simulink model "LKAS_AutoSave_20220223_1234"  (R2018b)
settings: Solver=FixedStepDiscrete  StartTime=0.0  StopTime=10.0  FixedStep=0.01  RelTol=1e-3
InitFcn:
  | tmpVer = ver('MATLAB');
  | tmpVer = str2num(tmpVer.Version);
  | % -------------------------------------------------------------------
  | %  MATLAB file generated by Simulink.saveVars on 21-Nov-2019 10:06:14
  | %  MATLAB version: 7.13.0.564 (R2011b)
  | % -------------------------------------------------------------------
  | 
  | 
  | SInt16 = Simulink.AliasType;
  | SInt16.Description = 'Num';
  | if (tmpVer > 7.11)
  | 	SInt16.DataScope = 'Auto';
  | end
  | SInt16.HeaderFile = 'Rte_Type.h';
  | SInt16.BaseType = 'int16';
  | 
  | SInt32 = Simulink.AliasType;
  | SInt32.Description = 'Num';
  | if (tmpVer > 7.11)
  | 	SInt32.DataScope = 'Auto';
  | end
  | SInt32.HeaderFile = 'Rte_Type.h';
  | SInt32.BaseType = 'int32';
  | 
  | SInt8 = Simulink.AliasType;
  | SInt8.Description = 'Num';
  | if (tmpVer > 7.11)
  | 	SInt8.DataScope = 'Auto';
  | end
  | SInt8.HeaderFile = 'Rte_Type.h';
  | SInt8.BaseType = 'int8';
  | 
  | T_A_m2_1024_1_u32 = Simulink.NumericType;
  | T_A_m2_1024_1_u32.Description = 'm2 (square meters  (m2))';
  | if (tmpVer > 7.11)
  | 	T_A_m2_1024_1_u32.DataScope = 'Auto';
  | end
  | T_A_m2_1024_1_u32.HeaderFile = 'Rte_Type.h';
  | T_A_m2_1024_1_u32.DataTypeMode = 'Fixed-point: slope and bias scaling';
  | T_A_m2_1024_1_u32.SignednessBool = false;
  | T_A_m2_1024_1_u32.WordLength = 32;
  | T_A_m2_1024_1_u32.FixedExponent = -10;
  | T_A_m2_1024_1_u32.SlopeAdjustmentFactor = 1;
  | T_A_m2_1024_1_u32.Bias = 0;
  | T_A_m2_1024_1_u32.DataTypeOverride = 'Inherit';
  | T_A_m2_1024_1_u32.IsAlias = true;
  | 
  | T_A_m2_65536_1_u16 = Simulink.NumericType;
  | T_A_m2_65536_1_u16.Description = 'm2 (square meters  (m2))';
  | if (tmpVer > 7.11)
  | 	T_A_m2_65536_1_u16.DataScope = 'Auto';
  | end
  | T_A_m2_65536_1_u16.HeaderFile = 'Rte_Type.h';
  | T_A_m2_65536_1_u16.DataTypeMode = 'Fixed-point: slope and bias scaling';
  | T_A_m2_65536_1_u16.SignednessBool = false;
  | T_A_m2_65536_1_u16.WordLength = 16;
  | T_A_m2_65536_1_u16.FixedExponent = -16;
  | T_A_m2_65536_1_u16.SlopeAdjustmentFactor = 1;
  | T_A_m2_65536_1_u16.Bias = 0;
  | T_A_m2_65536_1_u16.DataTypeOverride = 'Inherit';
  | ... (+4647 lines)
StopFcn:
  | clear  T_A_m2_1024_1_u32 T_A_m2_65536_1_u16 T_A_m2_Float32 T_A_mm2_10_1_u16 T_A_mm2_4_1_s16 T_A_mm2_Float32 T_Cnt_Num_10_1_u32 T_Cnt_Num_1_1_s16 T_Cnt_Num_1_1_s32 T_Cnt_Num_1_1_s8 T_Cnt_Num_1_1_u16 T_Cnt_Num_1_1_u32 T_Cnt_Num_1_1_u8 T_E_J_1_1_s32 T_E_J_Float32 T_E_kJ_128_1_s32 T_E_kJ_Float32 T_E_kwh_10_1_u16 T_E_kwh_Float32 T_Epl_kwhpkm_100_1_u16 T_Epl_kwhpkm_Float32 T_F_N_1_1_s16 T_F_N_Float32 T_I_A_1000_1_u16 T_I_A_1048576_1_s32 T_I_A_2048_1_s16 T_I_A_32_1_s16 T_I_A_Float32 T_I_mA_1_1_s16 T_I_mA_32768_128_s16 T_I_mA_Float32 T_J_kgpm2_128_1_u16 T_J_kgpm2_Float32 T_K_NA_1000_1_s16 T_K_NA_100_1_s16 T_K_NA_100_1_u16 T_K_NA_1024_1_s16 T_K_NA_1024_1_u16 T_K_NA_128_1_s16 T_K_NA_128_1_u16 T_K_NA_128_1_u8 T_K_NA_16777216_1_u32 T_K_NA_16_1_s16 T_K_NA_16_1_u16 T_K_NA_16_1_u8 T_K_NA_1_16_u16 T_K_NA_1_1_s16 T_K_NA_1_1_u16 T_K_NA_1_1_u8 T_K_NA_32768_1_s16 T_K_NA_32768_1_u16 T_K_NA_32_1_s8 T_K_NA_4096_1_u16 T_K_NA_4194304_1_s32 T_K_NA_4194304_1_u16 T_K_NA_65536_1_s32 T_K_NA_65536_1_u16 T_K_NA_8192_1_s16 T_K_NA_8_1_s16 T_K_NA_Float32 T_M_Nm_16_1_s16 T_M_Nm_1_1_s16 T_M_Nm_32768_1_s16 T_M_Nm_32_1_s16 T_M_Nm_4_1_s16 T_M_Nm_512_1_s16 T_M_Nm_Float32 T_P_W_1_4_s16 T_P_W_1_8_s16 T_P_W_Float32 T_P_kW_128_1_s16 T_P_kW_1_8_s16 T_P_kW_8_1_s32 T_P_kW_Float32 T_Pct_pct_1024_1_s32 T_Pct_pct_1024_1_u32 T_Pct_pct_10_1_s16 T_Pct_pct_10_1_u32 T_Pct_pct_128_100_s8 T_Pct_pct_1_1_s16 T_Pct_pct_1_4_u8 T_Pct_pct_255_100_u16 T_Pct_pct_255_100_u8 T_Pct_pct_256_1_s16 T_Pct_pct_256_1_u16 T_Pct_pct_65535_100_u16 T_Pct_pct_Float32 T_R_ohm_1024_1_s16 T_R_ohm_32_1_s16 T_R_ohm_Float32 T_TK_K_16_1_s16 T_TK_K_Float32 T_T_degC_10_400_1_u16 T_T_degC_16_1_s16 T_T_degC_1_40_1_u8 T_T_degC_2_80_1_u8 T_T_degC_Float32 T_U_V_1000_1_u16 T_U_V_10_1_u8 T_U_V_200_1_u8 T_U_V_32_1_s16 T_U_V_4096_1_s16 T_U_V_512_1_s16 T_U_V_65535_8_u16 T_U_V_8192_1_u16 T_U_V_Float32 T_U_mV_1_1_s16 T_U_mV_256_20_u16 T_U_mV_Float32 T_V_l_256_1_s16 T_V_l_4096_1_s16 T_V_l_64_1_s16 T_V_l_65535_100_u16 T_V_l_Float32 T_V_ml_128_1_s16 T_V_ml_1_1_s16 T_V_ml_32768_1_s16 T_V_ml_Float32 T_V_ul_32_1_u16 T_V_ul_Float32 T_Vpl_clpkm_512_1_u16 T_Vpl_clpkm_Float32 T_a_kphps_16_1_s16 T_a_kphps_Float32 T_a_mps2_128_1_s16 T_a_mps2_Float32 T_c_MJpkg_256_1_s16 T_c_MJpkg_Float32 T_c_kJpgpK_1024_1_s16 T_c_kJpgpK_Float32 T_c_kJpkgpK_128_1_u16 T_c_kJpkgpK_Float32 T_chrg_Ah_1_1_s16 T_chrg_Ah_1_1_u16 T_chrg_Ah_1_1_u8 T_chrg_Ah_256_1_u16 T_chrg_Ah_4194304_1_s32 T_chrg_Ah_512_1_u16 T_chrg_Ah_8_1_u16 T_chrg_Ah_Float32 T_cmp_NA_100_1_s16 T_cmp_NA_128_1_s16 T_cmp_NA_16_1_s16 T_cmp_NA_32768_1_u16 T_cmp_NA_Float32 T_d2n_rpmps2_4_1_s16 T_d2n_rpmps2_Float32 T_dPct_pctps_16_1_s16 T_dPct_pctps_256_1_s16 T_dPct_pctps_Float32 T_dT_degCps_128_1_s16 T_dT_degCps_Float32 T_dV_lph_1_1_s16 T_dV_lph_Float32 T_dV_lpm_128_1_s16 T_dV_lpm_32_1_s16 T_dV_lpm_Float32 T_dV_lps_1024_1_u16 T_dV_lps_4_1_u16 T_dV_lps_Float32 T_dV_mlps_1024_1_s16 T_dV_mlps_Float32 T_d_BitField16 T_dm_gps_128_1_s16 T_dm_gps_128_1_u16 T_dm_gps_256_1_u16 T_dm_gps_Float32 T_dm_mgps_1_1_s16 T_dm_mgps_Float32 T_dn_rpmps_1_1_s16 T_dn_rpmps_2_1_s16 T_dn_rpmps_Float32 T_dp_Paps_1_1_s16 T_dp_Paps_Float32 T_dp_kPaps_1_1_s16 T_dp_kPaps_8_1_s16 T_dp_kPaps_Float32 T_dphi_degps_128_1_s16 T_dphi_degps_8_1_s16 T_dphi_degps_Float32 T_dr_ps_256_1_s16 T_dr_ps_Float32 T_drho_mgplps_1_2_s16 T_drho_mgplps_Float32 T_e_NA_1_1_u8 T_f_Hz_1_1_u16 T_f_Hz_1_1_u32 T_f_Hz_64_1_u16 T_f_Hz_8_1_s16 T_f_Hz_Float32 T_g_BitField32 T_l_km_16_1_s16 T_l_km_1_1_u16 T_l_km_1_1_u32 T_l_km_Float32 T_l_m_1024_1_s16 T_l_m_16_1_s16 T_l_m_1_1_u32 T_l_m_Float32 T_l_mm_16_1_s16 T_l_mm_1_1_u16 T_l_mm_4096_1_s16 T_l_mm_4_1_u8 T_l_mm_64_1_s16 T_l_mm_Float32 T_m_g_1_1_s16 T_m_g_2048_1_s16 T_m_g_32_1_u16 T_m_g_Float32 T_m_kg_1024_1_s16 T_m_kg_1_1_s16 T_m_kg_1_1_u32 T_m_kg_Float32 T_m_mg_128_1_s16 T_m_mg_32_1_s16 T_m_mg_Float32 T_n_rpm_1_1_s16 T_n_rpm_1_25_u8 T_n_rpm_256_50_u16 T_n_rpm_2_25_u8 T_n_rpm_4_1_u16 T_n_rpm_Float32 T_p_MPa_64_1_s16 T_p_MPa_Float32 T_p_Pa_1_1_s16 T_p_Pa_Float32 T_p_kPa_1_10_u16 T_p_kPa_1_1_s16 T_p_kPa_1_1_u8 T_p_kPa_256_1_u16 T_p_kPa_32_1_u16 T_p_kPa_64_1_s16 T_p_kPa_Float32 T_phi_deg_100_1_s16 T_phi_deg_1024_1_s16 T_phi_deg_128_1_s16 T_phi_deg_1_1_u8 T_phi_deg_256_1_s16 T_phi_deg_2_1_s8 T_phi_deg_32_1_s16 T_phi_deg_512_6_s32 T_phi_deg_Float32 T_phi_rad_2048_1_s16 T_phi_rad_Float32 T_r_NA_1024_1_s16 T_r_NA_1024_1_u16 T_r_NA_16384_1_s16 T_r_NA_16_1_s16 T_r_NA_256_1_s8 T_r_NA_256_1_u16 T_r_NA_32768_1_u16 T_r_NA_32_1_u16 T_r_NA_4096_1_s16 T_r_NA_65535_2_u16 T_r_NA_8192_1_u16 T_r_NA_Float32 T_rho_gpl_8192_1_s16 T_rho_gpl_Float32 T_rho_kgpm3_16_1_s16 T_rho_kgpm3_Float32 T_rho_mgpl_1_1_s16 T_rho_mgpl_64_1_s16 T_rho_mgpl_Float32 T_t_hour_1_1_s16 T_t_hour_Float32 T_t_m_1_1_u16 T_t_m_Float32 T_t_ms_1_1_s16 T_t_ms_1_1_u16 T_t_ms_1_1_u32 T_t_ms_4096_1_s16 T_t_ms_64_1_s16 T_t_ms_Float32 T_t_s_1000_1_s16 T_t_s_100_1_s16 T_t_s_10_1_s16 T_t_s_10_1_u16 T_t_s_1_1_s16 T_t_s_1_1_u16 T_t_s_1_1_u32 T_t_s_Float32 T_t_us_10_1_u32 T_t_us_1_1_s16 T_t_us_1_1_u32 T_t_us_1_4_u16 T_t_us_Float32 T_v_kph_1_1_u8 T_v_kph_64_1_s16 T_v_kph_64_1_u16 T_v_kph_Float32 T_v_mps_256_1_s16 T_v_mps_Float32 T_w_radps_32_1_s16 T_w_radps_Float32 T_y_BitField8 T_y_BitFieldDiagProgress T_y_BitFieldDiagStatus T_y_NA_1_1_u8 SInt16 SInt32 SInt8 T_BOOLEAN UInt16 UInt32 UInt8 s16 s32 s8 u16 u32 u8
model workspace (MAT data in the model file):
  MCOS : class17 (value not decoded)
  MCOS : class17 (value not decoded)
  MCOS : class17 (value not decoded)
  MCOS : class17 (value not decoded)
  MCOS : class17 (value not decoded)
  MCOS : class17 (value not decoded)
  MCOS : class17 (value not decoded)
  MCOS : class17 (value not decoded)
  MCOS : class17 (value not decoded)
  MCOS : class17 (value not decoded)
  MCOS : class17 (value not decoded)
  MCOS : class17 (value not decoded)
  MCOS : class17 (value not decoded)
  MCOS : class17 (value not decoded)
  MCOS : class17 (value not decoded)
  MCOS : class17 (value not decoded)
  MCOS : class17 (value not decoded)
  MCOS : class17 (value not decoded)
  MCOS : class17 (value not decoded)
  MCOS : class17 (value not decoded)
  MCOS : class17 (value not decoded)
  MCOS : class17 (value not decoded)
  MCOS : class17 (value not decoded)
  MCOS : class17 (value not decoded)
  MCOS : class17 (value not decoded)
  MCOS : class17 (value not decoded)
  MCOS : class17 (value not decoded)
  MCOS : class17 (value not decoded)
  MCOS : class17 (value not decoded)
  MCOS : class17 (value not decoded)
  MCOS : class17 (value not decoded)
  MCOS : class17 (value not decoded)
  MCOS : class17 (value not decoded)
  MCOS : class17 (value not decoded)
  MCOS : class17 (value not decoded)
  MCOS : class17 (value not decoded)
  MCOS : class17 (value not decoded)
  MCOS : class17 (value not decoded)
  MCOS : class17 (value not decoded)
  MCOS : class17 (value not decoded)
  MCOS : class17 (value not decoded)
  MCOS : class17 (value not decoded)
  MCOS : class17 (value not decoded)
  MCOS : class17 (value not decoded)
  MCOS : class17 (value not decoded)
  MCOS : class17 (value not decoded)
  MCOS : class17 (value not decoded)
  MCOS : class17 (value not decoded)
  MCOS : class17 (value not decoded)
  MCOS : class17 (value not decoded)
  MCOS : class17 (value not decoded)
  MCOS : class17 (value not decoded)
  MCOS : class17 (value not decoded)
  MCOS : class17 (value not decoded)
  MCOS : class17 (value not decoded)
  MCOS : class17 (value not decoded)
  MCOS : class17 (value not decoded)
  MCOS : class17 (value not decoded)
  MCOS : class17 (value not decoded)
  MCOS : class17 (value not decoded)
  MCOS : class17 (value not decoded)
  MCOS : class17 (value not decoded)
  MCOS : class17 (value not decoded)
  MCOS : class17 (value not decoded)
  MCOS : class17 (value not decoded)
  MCOS : class17 (value not decoded)
  MCOS : class17 (value not decoded)
  MCOS : class17 (value not decoded)
  MCOS : class17 (value not decoded)
  MCOS : class17 (value not decoded)
  MCOS : class17 (value not decoded)
  MCOS : class17 (value not decoded)
  MCOS : class17 (value not decoded)
  MCOS : class17 (value not decoded)
  MCOS : class17 (value not decoded)
  MCOS : class17 (value not decoded)
  MCOS : class17 (value not decoded)
  MCOS : class17 (value not decoded)
  MCOS : class17 (value not decoded)
  MCOS : class17 (value not decoded)
  MCOS : class17 (value not decoded)
  MCOS : class17 (value not decoded)
  MCOS : class17 (value not decoded)
  MCOS : class17 (value not decoded)
  MCOS : class17 (value not decoded)
  MCOS : class17 (value not decoded)
  MCOS : class17 (value not decoded)
  MCOS : class17 (value not decoded)
  MCOS : class17 (value not decoded)
  MCOS : class17 (value not decoded)
  MCOS : class17 (value not decoded)
  MCOS : class17 (value not decoded)
  MCOS : class17 (value not decoded)
  MCOS : class17 (value not decoded)
  MCOS : class17 (value not decoded)
  MCOS : class17 (value not decoded)
  MCOS : class17 (value not decoded)
  MCOS : class17 (value not decoded)
  MCOS : class17 (value not decoded)
  MCOS : class17 (value not decoded)
  MCOS : class17 (value not decoded)
  MCOS : class17 (value not decoded)
undefined symbols (not defined in the file): LKA_CarWidth, LKA_SampleTime, LKA_StrRatio_C, LKA_Veh2CamL_C, LKA_Veh2CamW_C, LKA_WhlBaseL_C, LL_CompHdAg_C, LL_CompSWA_C, LL_CrvtPrvwT_C, LL_DesDvt_C, LL_DvtComp_C, LL_DvtPrvwT_C, LL_DvtSpdDet_vDvtSpdMin_C, LL_HandsOff_ExitTime, LL_HandsOff_TextTime, LL_HandsOff_WarnTime, LL_HdAgExT_C, LL_HdAgPrvwT_C, LL_LAccMax_C, LL_LAccRMax_C, LL_LDW_EarliestWarnLine_C, LL_LDW_LatestWarnLine_C, LL_LDWS_SUPPRESS_HEADING, LL_LFClb_TFC_FfCtlRatio_C, LL_LFClb_TFC_KdBalance_C, LL_LFClb_TFC_KdMaxSWA_C, LL_LFClb_TFC_KdV1_C, LL_LFClb_TFC_KdV2_C, LL_LFClb_TFC_KdVehSpdLwr_C, LL_LFClb_TFC_KdVehSpdUpr_C, LL_LFClb_TFC_Ki_C, LL_LFClb_TFC_KiMaxSWA_C, LL_LFClb_TFC_Kp_C, LL_LFClb_TFC_KpKlat_C, LL_LFClb_TFC_KpV1_C, LL_LFClb_TFC_KpV2_C, LL_LFClb_TFC_KpVehSpdLwr_C, LL_LFClb_TFC_KpVehSpdUpr_C, LL_LFClb_TFC_PrvwT_C, LL_LKA_EarliestWarnLine_C, LL_LKA_LatestWarnLine_C, LL_LKAExPrcs_ExitC0Dvt, LL_LKAExPrcs_ExitC0Swt, LL_LKAExPrcs_tiExitTime1, LL_LKAExPrcs_tiExitTime2, LL_LKAExPrcs_tiExitTime3, LL_LKAS_OUT_OF_CONTROL_LAT_VEL, LL_LKAS_OUT_OF_CONTROL_TTLC, LL_LKASWASyn_M0, LL_LKASWASyn_M1, LL_LKASWASyn_M2, LL_LKASWASyn_M3K, LL_LKASWASyn_SWAaddMax, LL_LKASWASyn_T2, LL_LKASWASyn_tiTrqSwaRtTime, LL_LKASWASyn_tiTrqSwaTime, LL_LKASWASyn_TrqMax, LL_LKASWASyn_TrqSwaAddSwt, LL_LKASWASyn_TrqSwaRateDiff, LL_LSpdCompT_C ... (+43)
libraries: simulink x138, canmsglib x8, dspstat3 x3, simulink_extras x1
(part 10 of 20)

== system LKAS_AutoSave_20220223_1234/LKAS/LL/LLOn/LKA/Lane Following (LF)/Preview Information Calculation (PIC) ==
  PIC_bsLKAInPInfo : Inport
  Bus Creator : BusCreator  Inputs=6
  Bus Selector1 : BusSelector  OutputSignals=bsPrDvtInfo.lPrvwDvtMean,bsPrHdAgInfo.phiPrvwHdAgMean,bsPrCrvtInfo.crPrvwCrvtMean,LaneWidth,bsPrHdAgInfo.PrvwZMean,bsPrCrvtInfo.crPrvwCrvtMean
  PIC_bsPrvwInfo : Outport
  wires:
  Bus Selector1/4 -> Bus Creator/4  "<LaneWidth>"
  Bus Creator/1 -> PIC_bsPrvwInfo/1
  PIC_bsLKAInPInfo/1 -> Bus Selector1/1
  Bus Selector1/3 -> Bus Creator/3  "<crPrvwCrvtMean>"
  Bus Selector1/2 -> Bus Creator/2  "<phiPrvwHdAgMean>"
  Bus Selector1/1 -> Bus Creator/1  "<lPrvwDvtMean>"
  Bus Selector1/5 -> Bus Creator/5  "<PrvwZMean>"
  Bus Selector1/6 -> Bus Creator/6  "<crPrvwCrvtMean>"

== system LKAS_AutoSave_20220223_1234/LKAS/LL/LLOn/LKA/Lane Following (LF)/Trajectory Following Control (TFC) ==
  TFC_bsPrvwInfo : Inport
  TFC_bsInInfoSyn : Inport  Port=2
  TFC_bsTFCClb : Inport  Port=3
  Bus Selector1 : BusSelector  OutputSignals=bsLKAClb.LL_TFCClb.LL_LFClb_TFC_PrvwT_C,bsLKAClb.LL_TFCClb.LL_LFClb_TFC_KpKlat_C,bsLKAClb.LL_TFCClb.LL_LFClb_TFC_KpVehSpdLwr_C,bsLKAClb.LL_TFCClb.LL_LFClb_TFC_KpVehSpdUpr_C,bsLKAClb.LL_TFCClb.LL_LFClb_TFC_KpV1_C,bsLKAClb.LL_TFCClb.LL_LFClb_TFC_KpV2_C,bsLKAClb.LL_TFCClb.LL_LFClb_TFC_Kp_C,bsLKAClb.LL_TFCClb.LL_LFClb_TFC_KiMaxSWA_C,bsLKAClb.LL_TFCClb.LL_LFClb_TFC_Ki_C,bsLKAClb.LL_TFCClb.LL_LFClb_TFC_KdMaxSWA_C,bsLKAClb.LL_TFCClb.LL_LFClb_TFC_KdBalance_C,bsLKAClb.LL_TFCClb.LL_LFClb_TFC_KdVehSpdLwr_C,bsLKAClb.LL_TFCClb.LL_LFClb_TFC_KdVehSpdUpr_C,bsLKAClb.LL_TFCClb.LL_LFClb_TFC_KdV1_C,bsLKAClb.LL_TFCClb.LL_LFClb_TFC_KdV2_C,bsConstantClb.LKA_CarWidth,bsLKAClb.LL_TFCClb.LL_LFClb_TFC_FfCtlRatio_C,bsConstantClb.LKA_WhlBaseL_C,bsConstantClb.LKA_StrRatio_C
  Bus Selector2 : BusSelector  OutputSignals=lPrvwDvtMean (signal 1),phiPrvwHdAgMean (signal 2),crPrvwCrvtMean (signal 3),LaneWidth (signal 4),PrvwZMean (signal 5),crPrvwCrvtMean (signal 6)
  Bus Selector3 : BusSelector  OutputSignals=bsLaneInfo.bsL0Info,bsLaneInfo.bsR0Info,bsVehMovInfo.ESC_VehSpd
  Feedback Control (FbCtl) : Subsystem
  Feedforward Control (FfCtl) : Subsystem
  TFC_phiFfSWACmd : Outport
  TFC_phiPropSWACmd : Outport  Port=2
  TFC_phiIntegSWACmd : Outport  Port=3
  TFC_phiDiffSWACmd : Outport  Port=4
  wires:
  Bus Selector1/16 -> Feedback Control (FbCtl)/25(FbCtl_CarWidth)  "<LKA_CarWidth>"
  Bus Selector2/4 -> Feedback Control (FbCtl)/7(FbCtl_LaneWidth)  "<LaneWidth (signal 4)>"
  Bus Selector1/15 -> Feedback Control (FbCtl)/24(FbCtl_KdV2_C)  "<LL_LFClb_TFC_KdV2_C>"
  Bus Selector1/14 -> Feedback Control (FbCtl)/23(FbCtl_KdV1_C)  "<LL_LFClb_TFC_KdV1_C>"
  Bus Selector1/13 -> Feedback Control (FbCtl)/22(FbCtl_KdVehSpdUpr_C)  "<LL_LFClb_TFC_KdVehSpdUpr_C>"
  Bus Selector1/12 -> Feedback Control (FbCtl)/21(FbCtl_KdVehSpdLwr_C)  "<LL_LFClb_TFC_KdVehSpdLwr_C>"
  Bus Selector1/7 -> Feedback Control (FbCtl)/16(FbCtl_Kp_C)  "<LL_LFClb_TFC_Kp_C>"
  Feedback Control (FbCtl)/3(FbCtl_phiFbDiffCtlSWA) -> TFC_phiDiffSWACmd/1
  Bus Selector3/2 -> Feedback Control (FbCtl)/2(FbCtl_bsR0Info)  "<bsR0Info>"
  Bus Selector3/1 -> Feedback Control (FbCtl)/1(FbCtl_bsL0Info)  "<bsL0Info>"
  TFC_bsInInfoSyn/1 -> Bus Selector3/1
  Bus Selector2/3 -> Feedforward Control (FfCtl)/3(FfCtl_crPrvwCrvt), Feedback Control (FbCtl)/6(FbCtl_PrvwCrvt)  "<crPrvwCrvtMean (signal 3)>"
  Feedforward Control (FfCtl)/1(FfCtl_phiFfSWA) -> TFC_phiFfSWACmd/1  "phiFfSWA"
  Feedback Control (FbCtl)/1(FbCtl_phiFbPropCtlSWA) -> TFC_phiPropSWACmd/1
  TFC_bsPrvwInfo/1 -> Bus Selector2/1  "bsPrvwInfo"
  Bus Selector2/1 -> Feedback Control (FbCtl)/4(FbCtl_PrvwDvt)  "<lPrvwDvtMean (signal 1)>"
  TFC_bsTFCClb/1 -> Bus Selector1/1
  Bus Selector1/1 -> Feedback Control (FbCtl)/10(FbCtl_PrvwT_C)  "<LL_LFClb_TFC_PrvwT_C>"
  Bus Selector1/2 -> Feedback Control (FbCtl)/11(FbCtl_KpKlat_C)  "<LL_LFClb_TFC_KpKlat_C>"
  Bus Selector3/3 -> Feedforward Control (FfCtl)/2(FfCtl_vVehSpd), Feedback Control (FbCtl)/3(FbCtl_VehSpd)  "<ESC_VehSpd>"
  Bus Selector1/3 -> Feedback Control (FbCtl)/12(FbCtl_KpVehSpdLwr_C)  "<LL_LFClb_TFC_KpVehSpdLwr_C>"
  Bus Selector1/4 -> Feedback Control (FbCtl)/13(FbCtl_KpVehSpdUpr_C)  "<LL_LFClb_TFC_KpVehSpdUpr_C>"
  Bus Selector1/5 -> Feedback Control (FbCtl)/14(FbCtl_KpV1_C1)  "<LL_LFClb_TFC_KpV1_C>"
  Bus Selector1/6 -> Feedback Control (FbCtl)/15(FbCtl_KpV2_C1)  "<LL_LFClb_TFC_KpV2_C>"
  Bus Selector1/17 -> Feedforward Control (FfCtl)/1(FfCtl_FfCtlRatio_C)  "<LL_LFClb_TFC_FfCtlRatio_C>"
  Bus Selector1/8 -> Feedback Control (FbCtl)/17(FbCtl_KiMaxSWA_C)  "<LL_LFClb_TFC_KiMaxSWA_C>"
  Bus Selector1/9 -> Feedback Control (FbCtl)/18(FbCtl_Ki_C)  "<LL_LFClb_TFC_Ki_C>"
  Feedback Control (FbCtl)/2(FbCtl_phiFbIntegCtlSWA) -> TFC_phiIntegSWACmd/1
  Bus Selector1/10 -> Feedback Control (FbCtl)/19(FbCtl_KdMaxSWA)  "<LL_LFClb_TFC_KdMaxSWA_C>"
  Bus Selector1/11 -> Feedback Control (FbCtl)/20(FbCtl_KdBalance)  "<LL_LFClb_TFC_KdBalance_C>"
  Bus Selector1/18 -> Feedforward Control (FfCtl)/4(FfCtl_lWhlBase_SY)  "<LKA_WhlBaseL_C>"
  Bus Selector1/19 -> Feedforward Control (FfCtl)/5(FfCtl_rTraRatio_C)  "<LKA_StrRatio_C>"
  Bus Selector2/2 -> Feedback Control (FbCtl)/5(FbCtl_PrvwHdAg)  "<phiPrvwHdAgMean (signal 2)>"
  Bus Selector2/5 -> Feedback Control (FbCtl)/8(PrvwZMean)  "<PrvwZMean (signal 5)>"
  Bus Selector2/6 -> Feedback Control (FbCtl)/9(PrvwCrvtMean)  "<crPrvwCrvtMean (signal 6)>"

== system LKAS_AutoSave_20220223_1234/LKAS/LL/LLOn/LKA/Plan To LaneFollowing (PTLF)/InsideJudge ==
  Flg : Inport
  Crvt : Inport  Port=2
  Compare To Constant : simulink/Logic and Bit Operations/Compare To Constant  relop===  const=1  OutDataTypeStr=boolean
  Compare To Constant1 : simulink/Logic and Bit Operations/Compare To Constant  relop===  const=2  OutDataTypeStr=boolean
  Constant : Constant  Value=0.001  OutDataTypeStr=single
  Constant3 : Constant  Value=-0.001  OutDataTypeStr=single
  Logical Operator : Logic  AllPortsSameDT=off  OutDataTypeStr=boolean
  Logical Operator1 : Logic  AllPortsSameDT=off  OutDataTypeStr=boolean
  Logical Operator2 : Logic  Operator=OR  AllPortsSameDT=off  OutDataTypeStr=boolean
  Relational Operator : RelationalOperator  OutDataTypeStr=boolean  RndMeth=Simplest
  Relational Operator1 : RelationalOperator  Operator=<=  OutDataTypeStr=boolean  RndMeth=Simplest
  Out1 : Outport
  wires:
  Compare To Constant/1 -> Logical Operator1/1  "LeftActive"
  Logical Operator1/1 -> Logical Operator2/1
  Logical Operator/1 -> Logical Operator2/2
  Flg/1 -> Compare To Constant1/1, Compare To Constant/1
  Relational Operator/1 -> Logical Operator/2  "RightCrvt"
  Compare To Constant1/1 -> Logical Operator/1  "RightActive"
  Constant/1 -> Relational Operator/2
  Relational Operator1/1 -> Logical Operator1/2  "LeftCrvt"
  Constant3/1 -> Relational Operator1/2
  Logical Operator2/1 -> Out1/1
  Crvt/1 -> Relational Operator1/1, Relational Operator/1

== system LKAS_AutoSave_20220223_1234/LKAS/LL/LLOn/LKA/Plan To LaneFollowing (PTLF)/InsideJudge1 ==
  Flg : Inport
  HdAgLft : Inport  Port=2
  HdAgRgt : Inport  Port=3
  T1 : Inport  Port=4
  Plan : Inport  Port=5
  Time : Inport  Port=6
  If : If  IfExpression=u1 == 1  ElseIfExpressions=u1 == 2
  If Action Subsystem : Subsystem  TreatAsAtomicUnit=on
  If Action Subsystem1 : Subsystem  TreatAsAtomicUnit=on
  If Action Subsystem2 : Subsystem  TreatAsAtomicUnit=on
  Merge : Merge  Inputs=3  InitialOutput=1
  Merge1 : Merge  Inputs=3  InitialOutput=0
  T1_1 : Outport
  Plan_1 : Outport  Port=2
  wires:
  Flg/1 -> If/1
  If/1 -> If Action Subsystem/Action
  If/2 -> If Action Subsystem1/Action
  If/3 -> If Action Subsystem2/Action
  HdAgLft/1 -> If Action Subsystem/3(HdAgLft)
  If Action Subsystem/1(T1_1) -> Merge/1
  If Action Subsystem1/1(T1_1) -> Merge/2
  If Action Subsystem2/1(T1_1) -> Merge/3
  If Action Subsystem/2(Plan_1) -> Merge1/1
  If Action Subsystem1/2(Plan_1) -> Merge1/2
  If Action Subsystem2/2(Plan_1) -> Merge1/3
  T1/1 -> If Action Subsystem/1(T1), If Action Subsystem1/1(T1), If Action Subsystem2/1(T1)
  Plan/1 -> If Action Subsystem/2(Plan), If Action Subsystem1/2(Plan), If Action Subsystem2/2(Plan)
  HdAgRgt/1 -> If Action Subsystem1/3(HdAgRgt)
  Merge/1 -> T1_1/1
  Merge1/1 -> Plan_1/1
  Time/1 -> If Action Subsystem1/4(Time), If Action Subsystem/4(Time)

== system LKAS_AutoSave_20220223_1234/LKAS/LL/LLOn/LKA/Plan To LaneFollowing (PTLF)/LowPass ==
  T : Inport
  u : Inport  Port=2
  dT : Inport  Port=3
  Add : Sum  Inputs=+-
  Add1 : Sum
  Add2 : Sum  OutDataTypeStr=single
  Divide : Product  Inputs=*/
  Divide1 : Product  Inputs=**
  Memory3 : Memory  InheritSampleTime=on
  SWACmdSyn_tiSmplT_C4 : Constant  OutDataTypeStr=single
  Saturation : Saturate  UpperLimit=50  LowerLimit=0
      settings: AttributesFormatString="Min = %<LowerLimit>  Max = %<UpperLimit>"
  Switch : Switch  Criteria=u2 > Threshold  Threshold=30
  Unit Delay : UnitDelay  SampleTime=-1
  y : Outport
  wires:
  Switch/1 -> Unit Delay/1, y/1
  Memory3/1 -> Add2/2
  Saturation/1 -> Memory3/1, Switch/2
  Add2/1 -> Saturation/1
  SWACmdSyn_tiSmplT_C4/1 -> Add2/1
  Add1/1 -> Switch/1
  Unit Delay/1 -> Add1/2, Add/2
  Divide1/1 -> Add1/1
  Add/1 -> Divide1/2
  Divide/1 -> Divide1/1
  u/1 -> Add/1, Switch/3
  dT/1 -> Divide/1
  T/1 -> Divide/2

== system LKAS_AutoSave_20220223_1234/LKAS/LL/LLOn/LKA/Plan To LaneFollowing (PTLF)/TickTime (TTime) ==
  Add2 : Sum  OutDataTypeStr=single
  Memory3 : Memory  InheritSampleTime=on
  Saturation : Saturate  UpperLimit=50  LowerLimit=0
      settings: AttributesFormatString="Min = %<LowerLimit>  Max = %<UpperLimit>"
  Out1 : Outport
  wires:
  Add2/1 -> Saturation/1
  Memory3/1 -> Add2/2
  Saturation/1 -> Out1/1, Memory3/1
  [LKA_SampleTime] -> Add2/1

== system LKAS_AutoSave_20220223_1234/LKAS/LL/LLOn/LKA/Plan To LaneFollowing (PTLF)/TimeGain ==
  Time : Inport
  T1 : Inport  Port=2
  TFC : Inport  Port=3
  Add1 : Sum
  Add2 : Sum  Inputs=+-
  Add3 : Sum  Inputs=-+
  Constant1 : Constant  Value=0  OutDataTypeStr=single
  Constant4 : Constant  OutDataTypeStr=single
  Divide : Product  Inputs=*/
  Divide8 : Product  Inputs=**
  Saturation4 : Saturate  UpperLimit=1  LowerLimit=0
      settings: AttributesFormatString="Min = %<LowerLimit>  Max = %<UpperLimit>"
  Out1 : Outport
  wires:
  Saturation4/1 -> Divide8/2
  Constant1/1 -> Add1/1, Add3/1
  Divide8/1 -> Add1/2
  Add1/1 -> Out1/1
  TFC/1 -> Divide/2
  T1/1 -> Add2/2
  Time/1 -> Add2/1
  Divide/1 -> Saturation4/1
  Add2/1 -> Divide/1
  Constant4/1 -> Add3/2
  Add3/1 -> Divide8/1

== system LKAS_AutoSave_20220223_1234/LKAS/LL/LLOn/LKA Input Processing (LKAInP)/Deviation Calculation (Dvt)/Left Front Conner Deviation Calculation (LFCDvtCalc) ==
  LFCDvtCalc_bsHdAgInfo : Inport
  LFCDvtCalc_lDvt : Inport  Port=2
  LFCDvtCalc_bsLLClb : Inport  Port=3
  Add1 : Sum  OutDataTypeStr=single
  Add5 : Sum  OutDataTypeStr=single
  Bus Selector : BusSelector  OutputSignals=bsConstantClb.LKA_Veh2CamW_C,bsConstantClb.LKA_Veh2CamL_C
  Cos2 : Trigonometry  Operator=cos
  Divide : Product  Inputs=**
  Divide1 : Product  Inputs=**
  Gain1 : Gain  Gain=-1  OutDataTypeStr=single
  Sin : Trigonometry
  DvtCalc_lLftDvt : Outport
  wires:
  LFCDvtCalc_lDvt/1 -> Add1/1
  Bus Selector/1 -> Add1/2  "<LKA_Veh2CamW_C>"
  LFCDvtCalc_bsLLClb/1 -> Bus Selector/1
  Bus Selector/2 -> Divide1/1  "<LKA_Veh2CamL_C>"
  LFCDvtCalc_bsHdAgInfo/1 -> Cos2/1, Sin/1
  Gain1/1 -> DvtCalc_lLftDvt/1
  Cos2/1 -> Divide/2
  Sin/1 -> Divide1/2
  Divide/1 -> Add5/1
  Divide1/1 -> Add5/2
  Add1/1 -> Divide/1
  Add5/1 -> Gain1/1

== system LKAS_AutoSave_20220223_1234/LKAS/LL/LLOn/LKA Input Processing (LKAInP)/Deviation Calculation (Dvt)/Right Front Conner Deviation Calculation (RFCDvtCalc) ==
  RFCDvtCalc_lDvt : Inport
  RFCDvtCalc_bsHdAgInfo : Inport  Port=2
  RFCDvtCalc_bsLLClb : Inport  Port=3
  Add1 : Sum  Inputs=+-  OutDataTypeStr=single
  Add5 : Sum  OutDataTypeStr=single
  Bus Selector1 : BusSelector  OutputSignals=bsConstantClb.LKA_Veh2CamW_C,bsConstantClb.LKA_Veh2CamL_C
  Cos2 : Trigonometry  Operator=cos
  Divide : Product  Inputs=**
  Divide1 : Product  Inputs=**
  Sin : Trigonometry
  DvtCalc_lRgtDvt : Outport
  wires:
  RFCDvtCalc_lDvt/1 -> Add1/1
  Bus Selector1/1 -> Add1/2  "<LKA_Veh2CamW_C>"
  Bus Selector1/2 -> Divide1/1  "<LKA_Veh2CamL_C>"
  Add5/1 -> DvtCalc_lRgtDvt/1
  Sin/1 -> Divide1/2
  Divide1/1 -> Add5/2
  RFCDvtCalc_bsHdAgInfo/1 -> Cos2/1, Sin/1
  Cos2/1 -> Divide/2
  Add1/1 -> Divide/1
  Divide/1 -> Add5/1
  RFCDvtCalc_bsLLClb/1 -> Bus Selector1/1

== system LKAS_AutoSave_20220223_1234/LKAS/LL/LLOn/LKA Input Processing (LKAInP)/Previewed Curvature Calculation (PrCrvt)/Curvature Ahead of Left Lane Line (CrvtAhdLft) ==
  CrvtAhdLft_bsL0Info : Inport
  CrvtAhdLft_lPrvwDstZ : Inport  Port=2
  Add : Sum  AccumDataTypeStr=single
  Bus Selector : BusSelector  OutputSignals=L0_C2,L0_C3
  Gain : Gain  Gain=2  OutDataTypeStr=single
  Gain1 : Gain  Gain=6  OutDataTypeStr=single
  Product : Product  OutDataTypeStr=single  RndMeth=Zero
  CrvtAhdLft_crCrvtAhdLft : Outport
  wires:
  Add/1 -> CrvtAhdLft_crCrvtAhdLft/1
  Product/1 -> Add/2
  Gain/1 -> Add/1
  Gain1/1 -> Product/1
  Bus Selector/1 -> Gain/1  "<L0_C2>"
  CrvtAhdLft_lPrvwDstZ/1 -> Product/2
  Bus Selector/2 -> Gain1/1  "<L0_C3>"
  CrvtAhdLft_bsL0Info/1 -> Bus Selector/1

== system LKAS_AutoSave_20220223_1234/LKAS/LL/LLOn/LKA Input Processing (LKAInP)/Previewed Curvature Calculation (PrCrvt)/Curvature Ahead of Left Lane Line (CrvtAhdLft)1 ==
  CrvtAhdRgt_lPrvwDstZ : Inport
  CrvtAhdRgt_bsR0Info : Inport  Port=2
  Add : Sum  AccumDataTypeStr=single
  Bus Selector : BusSelector  OutputSignals=R0_C2,R0_C3
  Gain : Gain  Gain=2  OutDataTypeStr=single
  Gain1 : Gain  Gain=6  OutDataTypeStr=single
  Product : Product  OutDataTypeStr=single  RndMeth=Zero
  CrvtAhdRgt_crCrvtAhdRgt : Outport
  wires:
  Add/1 -> CrvtAhdRgt_crCrvtAhdRgt/1
  Product/1 -> Add/2
  Gain/1 -> Add/1
  Gain1/1 -> Product/1
  Bus Selector/1 -> Gain/1  "<R0_C2>"
  CrvtAhdRgt_lPrvwDstZ/1 -> Product/2
  Bus Selector/2 -> Gain1/1  "<R0_C3>"
  CrvtAhdRgt_bsR0Info/1 -> Bus Selector/1

== system LKAS_AutoSave_20220223_1234/LKAS/LL/LLOn/LKA Input Processing (LKAInP)/Previewed Curvature Calculation (PrCrvt)/Lane Information Selection (LaneInfoSel) ==
  LaneInfoSel_stLKAActvFlg : Inport
  LaneInfoSel_facmLftLane : Inport  Port=2
  LaneInfoSel_facmRgtLane : Inport  Port=3
  If : If  IfExpression=u1==1  ElseIfExpressions=u1==2
  If Action Subsystem1 : Subsystem  TreatAsAtomicUnit=on
  If Action Subsystem2 : Subsystem  TreatAsAtomicUnit=on
  If Action Subsystem3 : Subsystem  TreatAsAtomicUnit=on
  Merge : Merge  Inputs=3
  LaneInfoSel_facmActvLane : Outport
  wires:
  If/3 -> If Action Subsystem3/Action
  If Action Subsystem3/1(Out1) -> Merge/3
  If Action Subsystem1/1(Out1) -> Merge/2
  If/2 -> If Action Subsystem1/Action
  Merge/1 -> LaneInfoSel_facmActvLane/1
  If Action Subsystem2/1(Out1) -> Merge/1
  If/1 -> If Action Subsystem2/Action
  LaneInfoSel_stLKAActvFlg/1 -> If/1
  LaneInfoSel_facmRgtLane/1 -> If Action Subsystem3/2(In2), If Action Subsystem1/1(In1)
  LaneInfoSel_facmLftLane/1 -> If Action Subsystem3/1(In1), If Action Subsystem2/1(In1)

== system LKAS_AutoSave_20220223_1234/LKAS/LL/LLOn/LKA Input Processing (LKAInP)/Previewed Curvature Calculation (PrCrvt)/Z Calculation (ZCalc) ==
  ZCalc_vVehSpd : Inport
  ZCalc_tiCrvtPrvwT_C : Inport  Port=2
  Divide : Product  Inputs=**  OutDataTypeStr=single
  kph to mps : Gain  Gain=1/3.6  OutDataTypeStr=single
  ZCalc_lPrvwDstZ : Outport
  wires:
  Divide/1 -> ZCalc_lPrvwDstZ/1
  kph to mps/1 -> Divide/1
  ZCalc_tiCrvtPrvwT_C/1 -> Divide/2
  ZCalc_vVehSpd/1 -> kph to mps/1

== system LKAS_AutoSave_20220223_1234/LKAS/LL/LLOn/LKA Input Processing (LKAInP)/Previewed Deviation Calculation (PrDvt)/Previewed Deviation of Left Lane Line (PrvwDvtLft) ==
  PrdcDvtLft_bsL0Info : Inport
  PrdcDvtLft_lPrvwDstZ : Inport  Port=2
  Add : Sum  Inputs=++++  AccumDataTypeStr=single
  Bus Selector : BusSelector  OutputSignals=L0_C0,L0_C1,L0_C2,L0_C3
  Product : Product  OutDataTypeStr=single  RndMeth=Zero
  Product3 : Product  OutDataTypeStr=single  RndMeth=Zero
  Product4 : Product  OutDataTypeStr=single  RndMeth=Zero
  Z*Z : Product  OutDataTypeStr=single  RndMeth=Zero
  Z*Z*Z : Product  OutDataTypeStr=single  RndMeth=Zero
  PrvwDvtLft_lPrvwDvtLft : Outport
  wires:
  Z*Z/1 -> Z*Z*Z/2, Product3/2
  Z*Z*Z/1 -> Product4/2
  Product4/1 -> Add/4
  Bus Selector/4 -> Product4/1  "<L0_C3>"
  Bus Selector/3 -> Product3/1  "<L0_C2>"
  Product3/1 -> Add/3
  Bus Selector/1 -> Add/1  "<L0_C0>"
  Product/1 -> Add/2
  Bus Selector/2 -> Product/1  "<L0_C1>"
  PrdcDvtLft_lPrvwDstZ/1 -> Z*Z/2, Product/2, Z*Z/1, Z*Z*Z/1
  PrdcDvtLft_bsL0Info/1 -> Bus Selector/1
  Add/1 -> PrvwDvtLft_lPrvwDvtLft/1

== system LKAS_AutoSave_20220223_1234/LKAS/LL/LLOn/LKA Input Processing (LKAInP)/Previewed Deviation Calculation (PrDvt)/Previewed Deviation of Right Lane Line (PrvwDvtRgt) ==
  PrdcDvtRgt_lPrvwDstZ : Inport
  PrdcDvtRgt_bsR0Info : Inport  Port=2
  Add : Sum  Inputs=++++  AccumDataTypeStr=single
  Bus Selector : BusSelector  OutputSignals=R0_C0,R0_C1,R0_C2,R0_C3
  Product : Product  OutDataTypeStr=single  RndMeth=Zero
  Product3 : Product  OutDataTypeStr=single  RndMeth=Zero
  Product4 : Product  OutDataTypeStr=single  RndMeth=Zero
  Z*Z : Product  OutDataTypeStr=single  RndMeth=Zero
  Z*Z*Z : Product  OutDataTypeStr=single  RndMeth=Zero
  PrvwDvtRgt_lPrvwDvtRgt : Outport
  wires:
  Z*Z/1 -> Z*Z*Z/2, Product3/2
  Z*Z*Z/1 -> Product4/2
  Product4/1 -> Add/4
  Bus Selector/4 -> Product4/1  "<R0_C3>"
  Bus Selector/3 -> Product3/1  "<R0_C2>"
  Product3/1 -> Add/3
  Bus Selector/1 -> Add/1  "<R0_C0>"
  Add/1 -> PrvwDvtRgt_lPrvwDvtRgt/1
  Product/1 -> Add/2
  Bus Selector/2 -> Product/1  "<R0_C1>"
  PrdcDvtRgt_lPrvwDstZ/1 -> Z*Z/2, Product/2, Z*Z/1, Z*Z*Z/1
  PrdcDvtRgt_bsR0Info/1 -> Bus Selector/1

== system LKAS_AutoSave_20220223_1234/LKAS/LL/LLOn/LKA Input Processing (LKAInP)/Previewed Deviation Calculation (PrDvt)/Z Calculation (ZCalc) ==
  ZCalc_vVehSpd : Inport
  ZCalc_tiDvtPrvwT_C : Inport  Port=2
  Divide : Product  Inputs=**  OutDataTypeStr=single
  kph to mps : Gain  Gain=1/3.6  OutDataTypeStr=single
  ZCalc_lPrvwDstZ : Outport
  wires:
  ZCalc_tiDvtPrvwT_C/1 -> Divide/2
  Divide/1 -> ZCalc_lPrvwDstZ/1
  kph to mps/1 -> Divide/1
  ZCalc_vVehSpd/1 -> kph to mps/1

== system LKAS_AutoSave_20220223_1234/LKAS/LL/LLOn/LKA Input Processing (LKAInP)/Previewed Heading Angle Calculation (PrHdAg)/Perdicted Heading Angle from Right Lane Line (PrdcHdAgRgt) ==
  PrdcHdAgRgt_lPrvwDstZ : Inport
  PrdcHdAgRgt_bsR0Info : Inport  Port=2
  Add : Sum  Inputs=+++  AccumDataTypeStr=single
  Bus Selector : BusSelector  OutputSignals=R0_C1,R0_C2,R0_C3
  Gain : Gain  Gain=2  OutDataTypeStr=single
  Gain1 : Gain  Gain=3  OutDataTypeStr=single
  Product3 : Product  OutDataTypeStr=single  RndMeth=Zero
  Product4 : Product  OutDataTypeStr=single  RndMeth=Zero
  Z*Z : Product  OutDataTypeStr=single  RndMeth=Zero
  PrdcHdAgRgt_phiPrdcHdAgRgt : Outport
  wires:
  Gain1/1 -> Product4/1
  Gain/1 -> Product3/1
  Z*Z/1 -> Product4/2
  Product4/1 -> Add/3
  Bus Selector/3 -> Gain1/1  "<R0_C3>"
  Bus Selector/2 -> Gain/1  "<R0_C2>"
  Product3/1 -> Add/2
  Bus Selector/1 -> Add/1  "<R0_C1>"
  PrdcHdAgRgt_lPrvwDstZ/1 -> Z*Z/2, Product3/2, Z*Z/1
  PrdcHdAgRgt_bsR0Info/1 -> Bus Selector/1
  Add/1 -> PrdcHdAgRgt_phiPrdcHdAgRgt/1

== system LKAS_AutoSave_20220223_1234/LKAS/LL/LLOn/LKA Input Processing (LKAInP)/Previewed Heading Angle Calculation (PrHdAg)/Perdicted Heading Angle from Right Lane Line (PrdcHdAgRgt)1 ==
  PrdcHdAgRgt_lPrvwDstZ : Inport
  PrdcHdAgRgt_bsR0Info : Inport  Port=2
  Add : Sum  Inputs=+++  AccumDataTypeStr=single
  Bus Selector : BusSelector  OutputSignals=R0_C1,R0_C2,R0_C3
  Gain : Gain  Gain=2  OutDataTypeStr=single
  Gain1 : Gain  Gain=3  OutDataTypeStr=single
  Product3 : Product  OutDataTypeStr=single  RndMeth=Zero
  Product4 : Product  OutDataTypeStr=single  RndMeth=Zero
  Z*Z : Product  OutDataTypeStr=single  RndMeth=Zero
  PrdcHdAgRgt_phiPrdcHdAgRgt : Outport
  wires:
  Gain1/1 -> Product4/1
  Gain/1 -> Product3/1
  Z*Z/1 -> Product4/2
  Product4/1 -> Add/3
  Bus Selector/3 -> Gain1/1  "<R0_C3>"
  Bus Selector/2 -> Gain/1  "<R0_C2>"
  Product3/1 -> Add/2
  Bus Selector/1 -> Add/1  "<R0_C1>"
  PrdcHdAgRgt_lPrvwDstZ/1 -> Z*Z/2, Product3/2, Z*Z/1
  PrdcHdAgRgt_bsR0Info/1 -> Bus Selector/1
  Add/1 -> PrdcHdAgRgt_phiPrdcHdAgRgt/1

== system LKAS_AutoSave_20220223_1234/LKAS/LL/LLOn/LKA Input Processing (LKAInP)/Previewed Heading Angle Calculation (PrHdAg)/Predicted Heading Angle from Left Lane Line (PrdcHdAgtLft) ==
  PrdcHdAgtLft_bsL0Info : Inport
  PrdcHdAgtLft_lPrvwDstZ : Inport  Port=2
  Add : Sum  Inputs=+++  AccumDataTypeStr=single
  Bus Selector : BusSelector  OutputSignals=L0_C1,L0_C2,L0_C3
  Gain : Gain  Gain=2  OutDataTypeStr=single
  Gain1 : Gain  Gain=3  OutDataTypeStr=single
  Product3 : Product  OutDataTypeStr=single  RndMeth=Zero
  Product4 : Product  OutDataTypeStr=single  RndMeth=Zero
  Z*Z : Product  OutDataTypeStr=single  RndMeth=Zero
  PrdcHdAgtLft_phiPrdcHdAgLft : Outport
  wires:
  Gain1/1 -> Product4/1
  Gain/1 -> Product3/1
  Z*Z/1 -> Product4/2
  Product4/1 -> Add/3
  Bus Selector/3 -> Gain1/1  "<L0_C3>"
  Bus Selector/2 -> Gain/1  "<L0_C2>"
  Product3/1 -> Add/2
  Bus Selector/1 -> Add/1  "<L0_C1>"
  PrdcHdAgtLft_lPrvwDstZ/1 -> Z*Z/2, Product3/2, Z*Z/1
  PrdcHdAgtLft_bsL0Info/1 -> Bus Selector/1
  Add/1 -> PrdcHdAgtLft_phiPrdcHdAgLft/1

== system LKAS_AutoSave_20220223_1234/LKAS/LL/LLOn/LKA Input Processing (LKAInP)/Previewed Heading Angle Calculation (PrHdAg)/Predicted Heading Angle from Left Lane Line (PrdcHdAgtLft)1 ==
  PrdcHdAgtLft_bsL0Info : Inport
  PrdcHdAgtLft_lPrvwDstZ : Inport  Port=2
  Add : Sum  Inputs=+++  AccumDataTypeStr=single
  Bus Selector : BusSelector  OutputSignals=L0_C1,L0_C2,L0_C3
  Gain : Gain  Gain=2  OutDataTypeStr=single
  Gain1 : Gain  Gain=3  OutDataTypeStr=single
  Product3 : Product  OutDataTypeStr=single  RndMeth=Zero
  Product4 : Product  OutDataTypeStr=single  RndMeth=Zero
  Z*Z : Product  OutDataTypeStr=single  RndMeth=Zero
  PrdcHdAgtLft_phiPrdcHdAgLft : Outport
  wires:
  Gain1/1 -> Product4/1
  Gain/1 -> Product3/1
  Z*Z/1 -> Product4/2
  Product4/1 -> Add/3
  Bus Selector/3 -> Gain1/1  "<L0_C3>"
  Bus Selector/2 -> Gain/1  "<L0_C2>"
  Product3/1 -> Add/2
  Bus Selector/1 -> Add/1  "<L0_C1>"
  PrdcHdAgtLft_lPrvwDstZ/1 -> Z*Z/2, Product3/2, Z*Z/1
  PrdcHdAgtLft_bsL0Info/1 -> Bus Selector/1
  Add/1 -> PrdcHdAgtLft_phiPrdcHdAgLft/1

== system LKAS_AutoSave_20220223_1234/LKAS/LL/LLOn/LKA Input Processing (LKAInP)/Previewed Heading Angle Calculation (PrHdAg)/Z Calculation (ZCalc) ==
  ZCalc_vVehSpd : Inport
  ZCalc_tiHdAgPrvwT_C : Inport  Port=2
  Divide : Product  Inputs=**  OutDataTypeStr=single
  kph to mps : Gain  Gain=1/3.6  OutDataTypeStr=single
  ZCalc_lPrvwDstZ : Outport
  wires:
  kph to mps/1 -> Divide/1
  Divide/1 -> ZCalc_lPrvwDstZ/1
  ZCalc_tiHdAgPrvwT_C/1 -> Divide/2
  ZCalc_vVehSpd/1 -> kph to mps/1

== system LKAS_AutoSave_20220223_1234/LKAS/LL/LLOn/LKA Input Processing (LKAInP)/Previewed Heading Angle Calculation (PrHdAg)/Z Calculation (ZCalc)1 ==
  ZCalc_vVehSpd : Inport
  ZCalc_tiHdAgPrvwT_C : Inport  Port=2
  Divide : Product  Inputs=**  OutDataTypeStr=single
  kph to mps : Gain  Gain=1/3.6  OutDataTypeStr=single
  ZCalc_lPrvwDstZ : Outport
  wires:
  kph to mps/1 -> Divide/1
  Divide/1 -> ZCalc_lPrvwDstZ/1
  ZCalc_tiHdAgPrvwT_C/1 -> Divide/2
  ZCalc_vVehSpd/1 -> kph to mps/1

== system LKAS_AutoSave_20220223_1234/LKAS/LL/LLOn/LKA Input Processing (LKAInP)/Steering Wheel Position Calculation (SWAPosCal)/Subsystem ==
  SWAIn : Inport
  LKA_SampleTime : Inport  Port=2
  Enable : EnablePort
      settings: AttributesFormatString=states = %<StatesWhenEnabling>
  Constant : Constant  Value=10  OutDataTypeStr=single
  LowPass : Subsystem
  Saturation : Saturate  UpperLimit=3  LowerLimit=-3
      settings: AttributesFormatString="Min = %<LowerLimit>  Max = %<UpperLimit>"
  SWAPos : Outport  InitialOutput=0
      settings: AttributesFormatString=%<OutputWhenDisabled> = %<InitialOutput>
  wires:
  SWAIn/1 -> LowPass/2(u)
  LowPass/1(y) -> Saturation/1  "SWAPos"
  Constant/1 -> LowPass/1(T)
  LKA_SampleTime/1 -> LowPass/3(dT)
  Saturation/1 -> SWAPos/1

== system LKAS_AutoSave_20220223_1234/LKAS/LL/LLOn/LKA Input Processing (LKAInP)/Steering Wheel Position Calculation (SWAPosCal)/Subsystem1 ==
  L0 : Inport
  R0 : Inport  Port=2
  VehSpd : Inport  Port=3
  SWA : Inport  Port=4
  LKA_SampleTime : Inport  Port=5
  Abs{2,4..7} (5 alike) : Abs
  Bus Selector : BusSelector  OutputSignals=L0_C1,L0_C2,L0_Q
  Bus Selector1 : BusSelector  OutputSignals=R0_C1,R0_C2,R0_Q
  Compare To Constant : simulink/Logic and Bit Operations/Compare To Constant  relop===  const=3.0  OutDataTypeStr=boolean
  Compare To Constant1 : simulink/Logic and Bit Operations/Compare To Constant  relop===  const=3.0  OutDataTypeStr=boolean
  Constant : Constant  Value=0.0001  OutDataTypeStr=single
  Constant1 : Constant  Value=0.005  OutDataTypeStr=single
  Constant3 : Constant  Value=2  OutDataTypeStr=single
  Constant4 : Constant  Value=50  OutDataTypeStr=single
  Constant5 : Constant  OutDataTypeStr=single
  Divide : Product  Inputs=*/
  Logical Operator : Logic  AllPortsSameDT=off  OutDataTypeStr=boolean
  Logical Operator1 : Logic  AllPortsSameDT=off  OutDataTypeStr=boolean
  Logical Operator3 : Logic  Inputs=5  AllPortsSameDT=off  OutDataTypeStr=boolean
  Logical Operator4 : Logic  AllPortsSameDT=off  OutDataTypeStr=boolean
  Relational Operator{,1..3,7} (5 alike) : RelationalOperator  Operator=<=  OutDataTypeStr=boolean  RndMeth=Simplest
  Relational Operator6 : RelationalOperator  OutDataTypeStr=boolean  RndMeth=Simplest
  Subsystem : Subsystem
  Flg : Outport
  wires:
  L0/1 -> Bus Selector/1
  R0/1 -> Bus Selector1/1
  Logical Operator1/1 -> Logical Operator3/1
  Bus Selector/3 -> Compare To Constant/1  "<L0_Q>"
  Abs2/1 -> Relational Operator7/1
  Bus Selector1/3 -> Compare To Constant1/1  "<R0_Q>"
  Relational Operator2/1 -> Logical Operator1/1
  Compare To Constant1/1 -> Logical Operator4/2
  Relational Operator6/1 -> Logical Operator3/4
  Abs7/1 -> Relational Operator3/1
  Constant1/1 -> Relational Operator3/2, Relational Operator2/2
  Constant/1 -> Relational Operator1/2, Relational Operator/2
  Abs4/1 -> Relational Operator/1
  Constant3/1 -> Divide/1
  Logical Operator3/1 -> Subsystem/Enable, Subsystem/1(In)  "SWA"
  VehSpd/1 -> Relational Operator6/1
  Constant4/1 -> Relational Operator6/2
  Abs6/1 -> Relational Operator2/1
  Compare To Constant/1 -> Logical Operator4/1
  Relational Operator7/1 -> Logical Operator3/5
  Bus Selector1/2 -> Abs5/1  "<R0_C2>"
  Abs5/1 -> Relational Operator1/1
  Relational Operator1/1 -> Logical Operator/2
  Relational Operator3/1 -> Logical Operator1/2
  SWA/1 -> Abs2/1
  Logical Operator/1 -> Logical Operator3/2
  Constant5/1 -> Relational Operator7/2
  Subsystem/1(Out) -> Flg/1
  Bus Selector/1 -> Abs6/1  "<L0_C1>"
  Bus Selector1/1 -> Abs7/1  "<R0_C1>"
  Logical Operator4/1 -> Logical Operator3/3
  Bus Selector/2 -> Abs4/1  "<L0_C2>"
  Divide/1 -> Subsystem/2(In1)
  Relational Operator/1 -> Logical Operator/1
  LKA_SampleTime/1 -> Divide/2

== system LKAS_AutoSave_20220223_1234/LKAS/LL/LLOn/LKA Input Processing (LKAInP)/Under The Limit (UndrLim)/Steering Wheel Angel Max (SWAMax) ==
  SWAMax_vVehSpd : Inport
  SWAMax_aLAcc_C : Inport  Port=2
  LKA_StrRatio_C : Inport  Port=3
  LKA_WhlBaseL_C : Inport  Port=4
  Constant : Constant  Value=0.09  OutDataTypeStr=single
  Divide1 : Product  Inputs=*/
  MATLAB Function : MATLAB Function  TreatAsAtomicUnit=on
  Saturation1 : Saturate  UpperLimit=0.0117  LowerLimit=0.00237
      settings: AttributesFormatString="Min = %<LowerLimit>  Max = %<UpperLimit>"
  Saturation3 : Saturate  UpperLimit=150  LowerLimit=60
      settings: AttributesFormatString="Min = %<LowerLimit>  Max = %<UpperLimit>"
  kph To mps : Gain  Gain=1/3.6  OutDataTypeStr=single
  SWAMax_phiSWAMax : Outport
  wires:
  LKA_StrRatio_C/1 -> MATLAB Function/3(i)
  LKA_WhlBaseL_C/1 -> MATLAB Function/4(L)
  kph To mps/1 -> MATLAB Function/1(v)
  SWAMax_vVehSpd/1 -> Saturation3/1, kph To mps/1
  Divide1/1 -> Saturation1/1
  Saturation1/1 -> MATLAB Function/5(K)
  SWAMax_aLAcc_C/1 -> MATLAB Function/2(ax)
  MATLAB Function/1(SWAmax) -> SWAMax_phiSWAMax/1
  Constant/1 -> Divide1/1
  Saturation3/1 -> Divide1/2  "Vx"

== system LKAS_AutoSave_20220223_1234/LKAS/LL/LLOn/LKA Input Processing (LKAInP)/Under The Limit (UndrLim)/Steering Wheel Angel Rate Max (SWARMax) ==
  SWARateMax_vVehSpd : Inport
  SWARateMax_aLAccR_C : Inport  Port=2
  LKA_StrRatio_C : Inport  Port=3
  LKA_WhlBaseL_C : Inport  Port=4
  Constant : Constant  Value=0.09  OutDataTypeStr=single
  Divide1 : Product  Inputs=*/
  MATLAB Function : MATLAB Function  TreatAsAtomicUnit=on
  Saturation1 : Saturate  UpperLimit=0.0117  LowerLimit=0.00237
      settings: AttributesFormatString="Min = %<LowerLimit>  Max = %<UpperLimit>"
  Saturation3 : Saturate  UpperLimit=150  LowerLimit=60
      settings: AttributesFormatString="Min = %<LowerLimit>  Max = %<UpperLimit>"
  kph To mps : Gain  Gain=1/3.6  OutDataTypeStr=single
  SWARMax_dphiSWARMax : Outport
  wires:
  kph To mps/1 -> MATLAB Function/1(v)
  LKA_WhlBaseL_C/1 -> MATLAB Function/4(L)
  LKA_StrRatio_C/1 -> MATLAB Function/3(i)
  MATLAB Function/1(SWARmax) -> SWARMax_dphiSWARMax/1
  SWARateMax_vVehSpd/1 -> Saturation3/1, kph To mps/1
  Divide1/1 -> Saturation1/1
  Saturation1/1 -> MATLAB Function/5(K)
  SWARateMax_aLAccR_C/1 -> MATLAB Function/2(dax)
  Constant/1 -> Divide1/1
  Saturation3/1 -> Divide1/2  "Vx"

== system LKAS_AutoSave_20220223_1234/LKAS/LL/LLOn/LL State Determination (LLStateDet)/LL State Machine Conditions (LLSMCon)/Activation Condition (ActvC) ==
  DACMode : Inport
  InInfoSyn : Inport  Port=2
  LKAInPInfo : Inport  Port=3
  LLClb : Inport  Port=4
  Activation Condition Synthesis (ActvCSyn) : Subsystem  Description=|
      | Block Name: Activation Condition Synthesis
      | Ab.: ActvCSyn
      | No.: 1.1.1.4.4
      | Rev: 0.0.1
      | Update Date: 19-3-26
  Bus Selector : BusSelector  OutputSignals=bsEPSInfo,bsLaneInfo.bsL0Info.L0_Q,bsLaneInfo.bsR0Info.R0_Q
  Bus Selector1 : BusSelector  OutputSignals=LaneWidth,bsDvtInfo.ILftDvt,bsDvtInfo.IRgtDvt
  Deviation Threshold Condition (DvtThresCon) : Subsystem
  EPS Controllability Enable Condition (EPSCtlEC) : Subsystem  Description=|
      | Block Name: EPS Controllability Enable Condition
      | Ab.: EPSCtlEC
      | No.: 1.1.1.4.1
      | Rev: 0.0.1
      | Update Date: 19-3-26
  Lane Quality Enable Condition (LaneQlEC) : Subsystem  Description=|
      | Block Name: Lane Quality Enable Condition
      | Ab.: LaneQlEC
      | No.: 1.1.1.4.3
      | Rev: 0.0.1
      | Update Date: 19-3-26
  ActvC_stLDWActvCSyn : Outport
  ActvC_stLKAActvCSyn : Outport  Port=2
  wires:
  InInfoSyn/1 -> Bus Selector/1, Deviation Threshold Condition (DvtThresCon)/5(DvtThresCon_InInfoSyn), Lane Quality Enable Condition (LaneQlEC)/1(LaneQlEC_InInfoSyn)
  Activation Condition Synthesis (ActvCSyn)/1(ActvCSyn_stLDWActvCSyn) -> ActvC_stLDWActvCSyn/1
  Deviation Threshold Condition (DvtThresCon)/2(DvtThresCon_stDvtThresActvFlgLKA) -> Activation Condition Synthesis (ActvCSyn)/4(ActvCSyn_stDvtThresActvFlgLKA), Lane Quality Enable Condition (LaneQlEC)/3(LaneQlEC_stDvtThresActvFlg)
  Bus Selector/1 -> EPS Controllability Enable Condition (EPSCtlEC)/1(EPSCtlEC_bsEPSInfo)  "<bsEPSInfo>"
  Bus Selector/2 -> Lane Quality Enable Condition (LaneQlEC)/4(LaneQlEC_stFacmL0Ql)  "<L0_Q>"
  Bus Selector/3 -> Lane Quality Enable Condition (LaneQlEC)/5(LaneQlEC_stFacmR0Ql)  "<R0_Q>"
  DACMode/1 -> Activation Condition Synthesis (ActvCSyn)/1(ActvCSyn_stDACMode)
  EPS Controllability Enable Condition (EPSCtlEC)/1(EPSCtlEC_stEPSCtlEC) -> Activation Condition Synthesis (ActvCSyn)/2(ActvCSyn_stEPSCtlEC)  "ACTIVE_EPS"
  Lane Quality Enable Condition (LaneQlEC)/1(LaneQlEC_stLaneQlECFlgLKA) -> Activation Condition Synthesis (ActvCSyn)/5(ActvCSyn_stLaneQlECFlg)  "ACTIVE_LANEQUALITY"
  Activation Condition Synthesis (ActvCSyn)/2(ActvCSyn_stLKAActvCSyn) -> ActvC_stLKAActvCSyn/1  "ACTIVE"
  LLClb/1 -> Deviation Threshold Condition (DvtThresCon)/4(DvtThresCon_bsDvtThresClb), Lane Quality Enable Condition (LaneQlEC)/2(LaneQlEC_SingleLane_Disable_Swt)
  Deviation Threshold Condition (DvtThresCon)/1(DvtThresCon_stDvtThresActvFlgLDW) -> Activation Condition Synthesis (ActvCSyn)/3(ActvCSyn_stDvtThresActvFlgLDW)
  LKAInPInfo/1 -> Bus Selector1/1
  Bus Selector1/2 -> Deviation Threshold Condition (DvtThresCon)/2(DvtThresCon_ILftDvt)  "<ILftDvt>"
  Bus Selector1/3 -> Deviation Threshold Condition (DvtThresCon)/3(DvtThresCon_IRgtDvt)  "<IRgtDvt>"
  Bus Selector1/1 -> Deviation Threshold Condition (DvtThresCon)/1(DvtThresCon_lLaneWidth)  "<LaneWidth>"

== system LKAS_AutoSave_20220223_1234/LKAS/LL/LLOn/LL State Determination (LLStateDet)/LL State Machine Conditions (LLSMCon)/Deactivation Condition (DeactvC) ==
  DACMode : Inport
  InInfoSyn : Inport  Port=2
  LKAInPInfo : Inport  Port=3
  LLClb : Inport  Port=4
  LLState : Inport  Port=5
  ExitFlg : Inport  Port=6
  Bus Selector : BusSelector  OutputSignals=bsVehMovInfo.ESC_VehSpd,bsEPSInfo
  Bus Selector1 : BusSelector  OutputSignals=LaneWidth,bsDvtInfo.ILftDvt,bsDvtInfo.IRgtDvt,bsPrCrvtInfo.crPrvwCrvt
  Deactivation Condition Synthesis (DeactvCSyn) : Subsystem  Description=|
      | Block Name: Deactivation Condition Synthesis
      | Ab.: DeactvCSyn
      | No.: 1.1.1.5.3
      | Rev: 0.0.1
      | Update Date: 19-3-26
  Deviation Threshold Condition (DvtThresCon) : Subsystem
  Driver Take Condition (DvrTkCon) : Subsystem  Description=|
      | Block Name: EPS Condition
      | Ab.: EPSC
      | No.: 1.1.1.5.2
      | Rev: 0.0.1
      | Update Date: 19-3-26
  EPS Condition (EPSC) : Subsystem  Description=|
      | Block Name: EPS Condition
      | Ab.: EPSC
      | No.: 1.1.1.5.2
      | Rev: 0.0.1
      | Update Date: 19-3-26
  DeactvC_stLDWDeactvCSyn : Outport
  DeactvC_stLKADeactvCSyn : Outport  Port=2
  wires:
  InInfoSyn/1 -> Bus Selector/1, Deviation Threshold Condition (DvtThresCon)/5(DvtThresCon_InInfoSyn)
  Deactivation Condition Synthesis (DeactvCSyn)/1(DeactvCSyn_stLDWDeactvCSyn) -> DeactvC_stLDWDeactvCSyn/1
  LLClb/1 -> EPS Condition (EPSC)/1(EPSC_bsLLClb), Driver Take Condition (DvrTkCon)/3(DvrTkCon_bsLLClb), Deviation Threshold Condition (DvtThresCon)/4(DvtThresCon_bsDvtThresClb)
  Deviation Threshold Condition (DvtThresCon)/2(DvtThresCon_stDvtThresActvFlgLKA) -> Driver Take Condition (DvrTkCon)/2(DvrTkCon_stActvFlg), Deactivation Condition Synthesis (DeactvCSyn)/3(DeactvCSyn_stDvtThresActvFlgLKA)
  LLState/1 -> EPS Condition (EPSC)/3(EPSC_bsLLState)
  Bus Selector/2 -> Driver Take Condition (DvrTkCon)/5(DvrTkCon_bsEPSInfo), EPS Condition (EPSC)/2(EPSC_bsEPSInfo)  "<bsEPSInfo>"
  EPS Condition (EPSC)/1(EPSC_stEPSCFlg) -> Deactivation Condition Synthesis (DeactvCSyn)/5(DeactvCSyn_stEPSCFlg)
  ExitFlg/1 -> Deactivation Condition Synthesis (DeactvCSyn)/6(DeactvCSyn_stExitFlg)
  DACMode/1 -> Deactivation Condition Synthesis (DeactvCSyn)/1(DeactvCSyn_stDACMode)
  Deactivation Condition Synthesis (DeactvCSyn)/2(DeactvCSyn_stLKADeactvCSyn) -> DeactvC_stLKADeactvCSyn/1  "DEACTIVE"
  Bus Selector/1 -> Driver Take Condition (DvrTkCon)/4(DvrTkCon_vVehSpd)  "<ESC_VehSpd>"
  Driver Take Condition (DvrTkCon)/1(DvrTkCon_stDvrTkConFlg) -> Deactivation Condition Synthesis (DeactvCSyn)/4(DvrTkCon_stDvrTkConFlg)
  LKAInPInfo/1 -> Bus Selector1/1
  Bus Selector1/3 -> Deviation Threshold Condition (DvtThresCon)/3(DvtThresCon_IRgtDvt)  "<IRgtDvt>"
  Bus Selector1/2 -> Deviation Threshold Condition (DvtThresCon)/2(DvtThresCon_ILftDvt)  "<ILftDvt>"
  Bus Selector1/4 -> Driver Take Condition (DvrTkCon)/1(DvrTkCon_crPrvwCrvt)  "<crPrvwCrvt>"
  Bus Selector1/1 -> Deviation Threshold Condition (DvtThresCon)/1(DvtThresCon_lLaneWidth)  "<LaneWidth>"
  Deviation Threshold Condition (DvtThresCon)/1(DvtThresCon_stDvtThresActvFlgLDW) -> Deactivation Condition Synthesis (DeactvCSyn)/2(DeactvCSyn_stDvtThresActvFlgLDW)
